simulink model "EX1_dys"  (R2023b)
settings: Solver=FixedStepDiscrete  StartTime=0.0  StopTime=0  RelTol=1e-3
libraries: CPOiS_SourcesSinks x10, CPOiS_DataManipulation x6
settings Model: Creator=alyskawa  LastModifiedBy=alyskawa

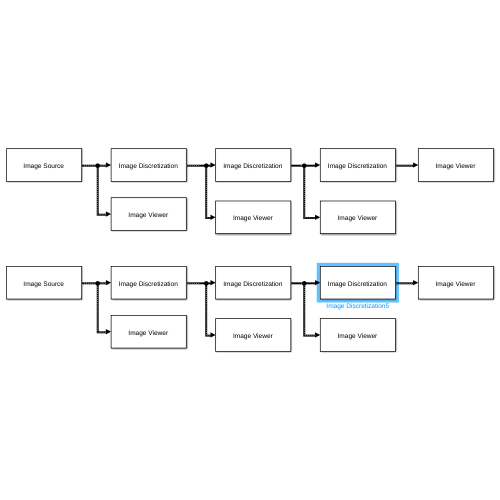
[thumbnail: Simulink's stored preview of the top-level diagram]
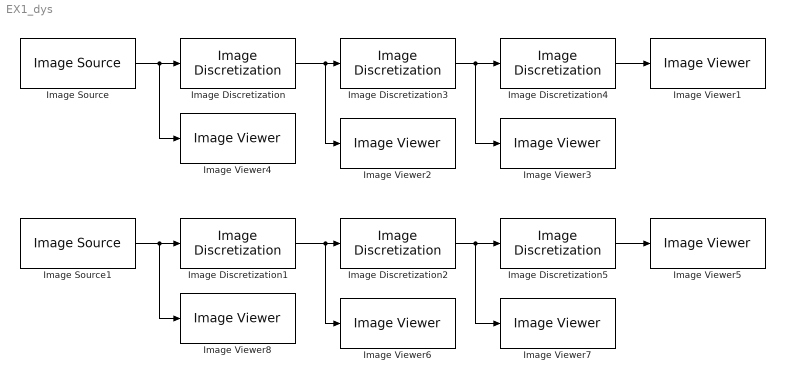
== system EX1_dys ==
  Image Discretization : CPOiS_DataManipulation/Image Discretization  factor=4
      settings: SourceProductName=CPOiS - Digital image and signal processing
  Image Discretization1 : CPOiS_DataManipulation/Image Discretization  factor=2
      settings: SourceProductName=CPOiS - Digital image and signal processing
  Image Discretization2 : CPOiS_DataManipulation/Image Discretization  factor=4
      settings: SourceProductName=CPOiS - Digital image and signal processing
  Image Discretization3 : CPOiS_DataManipulation/Image Discretization  factor=4
      settings: SourceProductName=CPOiS - Digital image and signal processing
  Image Discretization4 : CPOiS_DataManipulation/Image Discretization  factor=6
      settings: SourceProductName=CPOiS - Digital image and signal processing
  Image Discretization5 : CPOiS_DataManipulation/Image Discretization  factor=6
      settings: SourceProductName=CPOiS - Digital image and signal processing
  Image Source : CPOiS_SourcesSinks/Image Source  FileSelection=gull.png
      settings: SourceProductName=CPOiS - Digital image and signal processing
  Image Source1 : CPOiS_SourcesSinks/Image Source  FileSelection=ball.png
      settings: SourceProductName=CPOiS - Digital image and signal processing
  Image Viewer{1..8} (8 alike) : CPOiS_SourcesSinks/Image Viewer
      settings: SourceProductName=CPOiS - Digital image and signal processing
  wires:
  Image Source/1 -> Image Discretization/1, Image Viewer4/1
  Image Discretization/1 -> Image Viewer2/1, Image Discretization3/1
  Image Discretization4/1 -> Image Viewer1/1
  Image Discretization3/1 -> Image Viewer3/1, Image Discretization4/1
  Image Discretization1/1 -> Image Viewer6/1, Image Discretization2/1
  Image Source1/1 -> Image Discretization1/1, Image Viewer8/1
  Image Discretization5/1 -> Image Viewer5/1
  Image Discretization2/1 -> Image Viewer7/1, Image Discretization5/1
